simulink model "white_noise_whistle2"  (Simulink 7.3)
settings: Solver=ode3  StartTime=0.0  StopTime=1  FixedStep=1/11025  MaxStep=1/11025  MinStep=1/11025  RelTol=1e-3
libraries: simulink x1, simulink_extras x1
settings Model: Creator=Hörnstein  LastModifiedBy=Hörnstein
settings SolverCC: InitialStep=1/11025
settings OptimizationCC: InitFltsAndDblsToZero=on
settings DebuggingCC: AlgebraicLoopMsg=none  SaveWithParameterizedLinksMsg=none  SignalResolutionControl=TryResolveAllWithWarning  MultiTaskDSMMsg=warning  MultiTaskCondExecSysMsg=none
settings RTWCC: IncludeERTFirstTime=on
settings GRTTargetCC: TargetFcnLib=ansi_tfl_tmw.mat

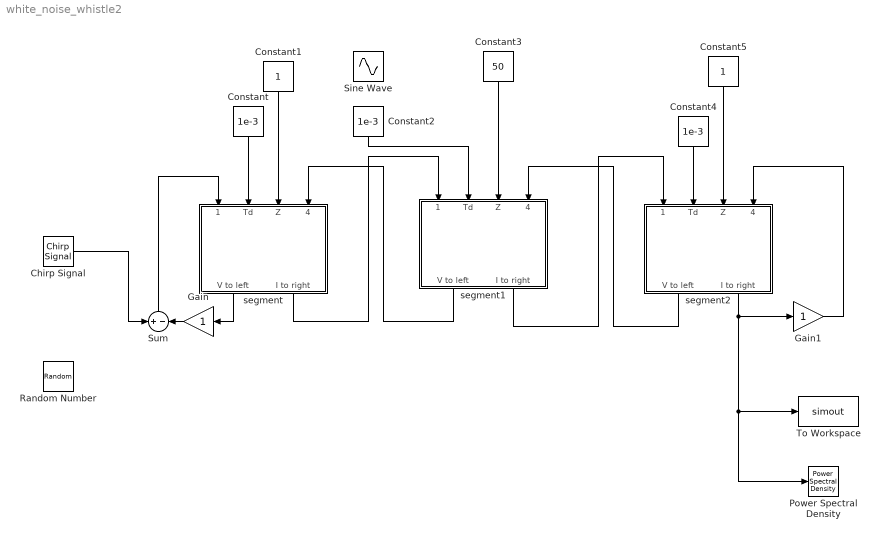
== system white_noise_whistle2 ==
  Chirp Signal : simulink/Sources/Chirp Signal  SystemSampleTime=-1  f1=0  T=1  f2=2000
  Constant : Constant  Value=1e-3  OutDataType=sfix(16)  OutScaling=2^0
  Constant1 : Constant  OutDataType=sfix(16)  OutScaling=2^0
  Constant2 : Constant  Value=1e-3  OutDataType=sfix(16)  OutScaling=2^0
  Constant3 : Constant  Value=50  OutDataType=sfix(16)  OutScaling=2^0
  Constant4 : Constant  Value=1e-3  OutDataType=sfix(16)  OutScaling=2^0
  Constant5 : Constant  OutDataType=sfix(16)  OutScaling=2^0
  Gain : Gain  ParameterDataType=sfix(16)  ParameterScaling=2^0  OutDataType=sfix(16)  OutScaling=2^0
  Gain1 : Gain  ParameterDataType=sfix(16)  ParameterScaling=2^0  OutDataType=sfix(16)  OutScaling=2^0
  Power Spectral Density : simulink_extras/Additional Sinks/Power Spectral Density  SystemSampleTime=-1  npts=1102  fftpts=1102  HowOften=64  sampleT=1/11025
  Random Number : RandomNumber  SampleTime=0
  Sine Wave : Sin  Amplitude=5e-4  Bias=6e-4  Frequency=2*pi  Phase=0  Samples=10  SampleTime=0  Offset=0
  Sum : Sum  Inputs=+|-  OutDataType=sfix(16)  OutScaling=2^0
  To Workspace : ToWorkspace  VariableName=simout  SampleTime=-1  SaveFormat=Array
  segment : Subsystem
  segment1 : Subsystem
  segment2 : Subsystem
  wires:
  Constant/1 -> segment/2(Td)
  Constant1/1 -> segment/3(Z)
  Sum/1 -> segment/1(I from left)
  segment1/1(V to left) -> segment/4(V from right)
  segment/2(I to right) -> segment1/1(I from left)
  Constant3/1 -> segment1/3(Z)
  segment2/1(V to left) -> segment1/4(V from right)
  segment1/2(I to right) -> segment2/1(I from left)
  Constant4/1 -> segment2/2(Td)
  Constant5/1 -> segment2/3(Z)
  segment2/2(I to right) -> Gain1/1, To Workspace/1, Power Spectral Density/1
  segment/1(V to left) -> Gain/1
  Gain/1 -> Sum/2
  Gain1/1 -> segment2/4(V from right)
  Constant2/1 -> segment1/2(Td)
  Chirp Signal/1 -> Sum/1

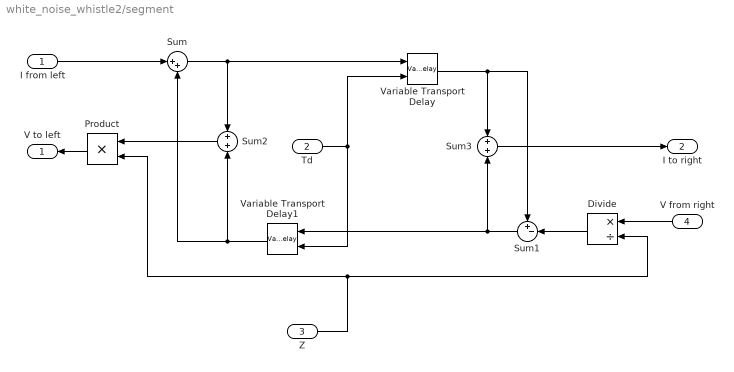
== system white_noise_whistle2/segment ==
  I from left : Inport  OutDataType=sfix(16)  OutScaling=2^0
  Td : Inport  Port=2  OutDataType=sfix(16)  OutScaling=2^0
  Z : Inport  Port=3  OutDataType=sfix(16)  OutScaling=2^0
  V from right : Inport  Port=4  OutDataType=sfix(16)  OutScaling=2^0
  Divide : Product  Inputs=*/  OutDataType=sfix(16)  OutScaling=2^-10
  Product : Product  OutDataType=sfix(16)  OutScaling=2^0  RndMeth=Zero
  Sum : Sum  Inputs=|++  OutDataType=sfix(16)  OutScaling=2^0
  Sum1 : Sum  Inputs=+-|  OutDataType=sfix(16)  OutScaling=2^0
  Sum2 : Sum  Inputs=+|+  OutDataType=sfix(16)  OutScaling=2^0
  Sum3 : Sum  Inputs=+|+  OutDataType=sfix(16)  OutScaling=2^0
  Variable Transport Delay : VariableTransportDelay  VariableDelayType=Variable transport delay  MaximumDelay=10
  Variable Transport Delay1 : VariableTransportDelay  VariableDelayType=Variable transport delay  MaximumDelay=10
  V to left : Outport  OutDataType=sfix(16)  OutScaling=2^0
  I to right : Outport  Port=2  OutDataType=sfix(16)  OutScaling=2^0
  wires:
  Sum3/1 -> I to right/1
  Product/1 -> V to left/1
  Z/1 -> Product/2, Divide/2
  Sum2/1 -> Product/1
  V from right/1 -> Divide/1
  I from left/1 -> Sum/1
  Divide/1 -> Sum1/2
  Variable Transport Delay/1 -> Sum1/1, Sum3/1
  Variable Transport Delay1/1 -> Sum/2, Sum2/2
  Sum/1 -> Variable Transport Delay/1, Sum2/1
  Sum1/1 -> Variable Transport Delay1/1, Sum3/2
  Td/1 -> Variable Transport Delay/2, Variable Transport Delay1/2

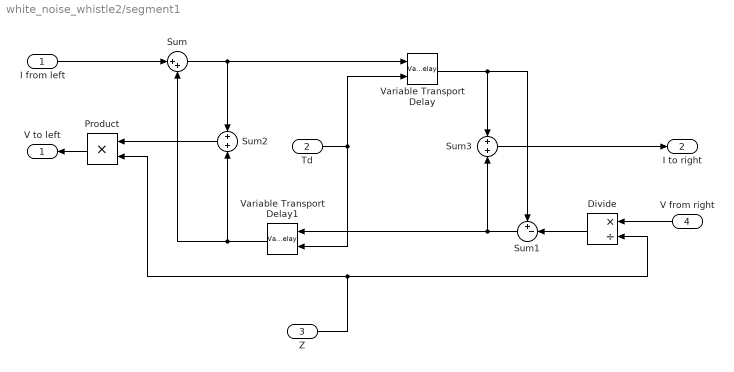
== system white_noise_whistle2/segment1 ==
  I from left : Inport  OutDataType=sfix(16)  OutScaling=2^0
  Td : Inport  Port=2  OutDataType=sfix(16)  OutScaling=2^0
  Z : Inport  Port=3  OutDataType=sfix(16)  OutScaling=2^0
  V from right : Inport  Port=4  OutDataType=sfix(16)  OutScaling=2^0
  Divide : Product  Inputs=*/  OutDataType=sfix(16)  OutScaling=2^-10
  Product : Product  OutDataType=sfix(16)  OutScaling=2^0  RndMeth=Zero
  Sum : Sum  Inputs=|++  OutDataType=sfix(16)  OutScaling=2^0
  Sum1 : Sum  Inputs=+-|  OutDataType=sfix(16)  OutScaling=2^0
  Sum2 : Sum  Inputs=+|+  OutDataType=sfix(16)  OutScaling=2^0
  Sum3 : Sum  Inputs=+|+  OutDataType=sfix(16)  OutScaling=2^0
  Variable Transport Delay : VariableTransportDelay  VariableDelayType=Variable transport delay  MaximumDelay=10
  Variable Transport Delay1 : VariableTransportDelay  VariableDelayType=Variable transport delay  MaximumDelay=10
  V to left : Outport  OutDataType=sfix(16)  OutScaling=2^0
  I to right : Outport  Port=2  OutDataType=sfix(16)  OutScaling=2^0
  wires:
  Sum3/1 -> I to right/1
  Product/1 -> V to left/1
  Z/1 -> Product/2, Divide/2
  Sum2/1 -> Product/1
  V from right/1 -> Divide/1
  I from left/1 -> Sum/1
  Divide/1 -> Sum1/2
  Variable Transport Delay/1 -> Sum1/1, Sum3/1
  Variable Transport Delay1/1 -> Sum/2, Sum2/2
  Sum/1 -> Variable Transport Delay/1, Sum2/1
  Sum1/1 -> Variable Transport Delay1/1, Sum3/2
  Td/1 -> Variable Transport Delay/2, Variable Transport Delay1/2

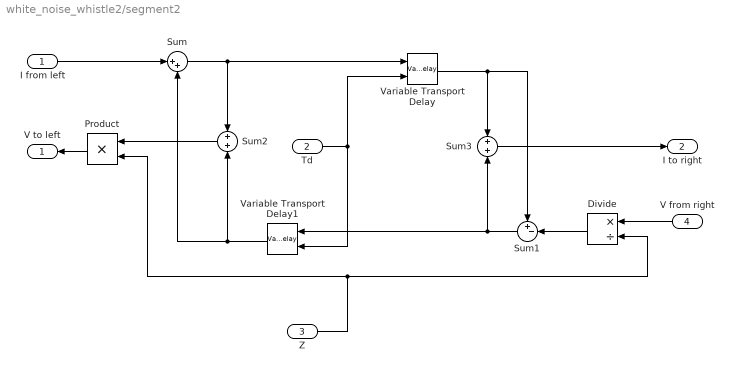
== system white_noise_whistle2/segment2 ==
  I from left : Inport  OutDataType=sfix(16)  OutScaling=2^0
  Td : Inport  Port=2  OutDataType=sfix(16)  OutScaling=2^0
  Z : Inport  Port=3  OutDataType=sfix(16)  OutScaling=2^0
  V from right : Inport  Port=4  OutDataType=sfix(16)  OutScaling=2^0
  Divide : Product  Inputs=*/  OutDataType=sfix(16)  OutScaling=2^-10
  Product : Product  OutDataType=sfix(16)  OutScaling=2^0  RndMeth=Zero
  Sum : Sum  Inputs=|++  OutDataType=sfix(16)  OutScaling=2^0
  Sum1 : Sum  Inputs=+-|  OutDataType=sfix(16)  OutScaling=2^0
  Sum2 : Sum  Inputs=+|+  OutDataType=sfix(16)  OutScaling=2^0
  Sum3 : Sum  Inputs=+|+  OutDataType=sfix(16)  OutScaling=2^0
  Variable Transport Delay : VariableTransportDelay  VariableDelayType=Variable transport delay  MaximumDelay=10
  Variable Transport Delay1 : VariableTransportDelay  VariableDelayType=Variable transport delay  MaximumDelay=10
  V to left : Outport  OutDataType=sfix(16)  OutScaling=2^0
  I to right : Outport  Port=2  OutDataType=sfix(16)  OutScaling=2^0
  wires:
  Sum3/1 -> I to right/1
  Product/1 -> V to left/1
  Z/1 -> Product/2, Divide/2
  Sum2/1 -> Product/1
  V from right/1 -> Divide/1
  I from left/1 -> Sum/1
  Divide/1 -> Sum1/2
  Variable Transport Delay/1 -> Sum1/1, Sum3/1
  Variable Transport Delay1/1 -> Sum/2, Sum2/2
  Sum/1 -> Variable Transport Delay/1, Sum2/1
  Sum1/1 -> Variable Transport Delay1/1, Sum3/2
  Td/1 -> Variable Transport Delay/2, Variable Transport Delay1/2
